simulink model "psc_gfl_parallel"  (R2023b)
settings: Solver=VariableStepAuto  StartTime=0.0  StopTime=1  RelTol=1e-3
values from neighbouring files (symbols this model uses):
  alpha_c = 2*pi*400    (= 2513.27412287)    [init.m]    (also in init_psc_parallel.m)
  f_sw = 10e3    (= 10000)    [init.m]    (also in init_psc_parallel.m)
  kpp = 3/2 * K^(-2)    (= 1.5)    [init.m]    (also in init_psc_parallel.m)
  L_f = 1e-3    (= 0.001)    [init.m]    (also in init_psc_parallel.m = 0.01)
  L_f1 = L_f    (= 0.001)    [init.m]    (also in init_psc_parallel.m = 0.01)
  L_f2 = L_f    (= 0.001)    [init.m]    (also in init_psc_parallel.m = 0.01)
  L_g = 2.5e-3    (= 0.0025)    [init.m]    (also in init_psc_parallel.m)
  R_a = 0.6    [init.m]    (also in init_psc_parallel.m = 0.32)
  R_L = 20    [init.m]    (also in init_psc_parallel.m)
  T_s = 1/(2*f_sw)    (= 5e-05)    [init.m]    (also in init_psc_parallel.m)
  U_dc = 48    [init.m]    (also in init_psc_parallel.m)
  u_gN = 24    [init.m]    (also in init_psc_parallel.m)
  w0_pll = 2*pi*20    (= 125.663706144)    [init.m]    (also in init_psc_parallel.m)
  w_b = 0.1*w_g    (= 31.4159265359)    [init.m]    (also in init_psc_parallel.m)
  w_g = 2*pi*50    (= 314.159265359)    [init.m]    (also in init_psc_parallel.m; psc_matlab.m = (P_ref - P)*K_p + w_1)
libraries: simulink x2
settings Model: Creator=maatt  LastModifiedBy=chowd
settings DataIOCC: ReturnWorkspaceOutputs=off

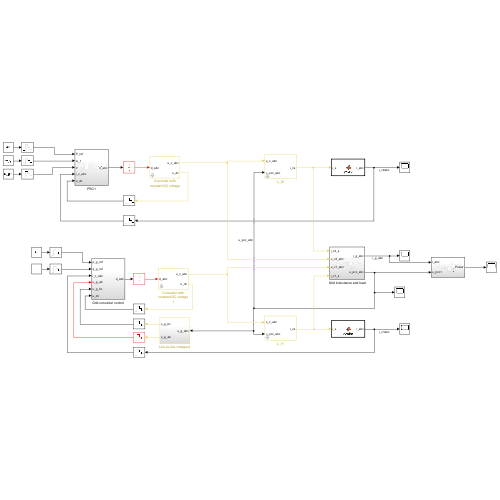
[thumbnail: Simulink's stored preview of the top-level diagram]
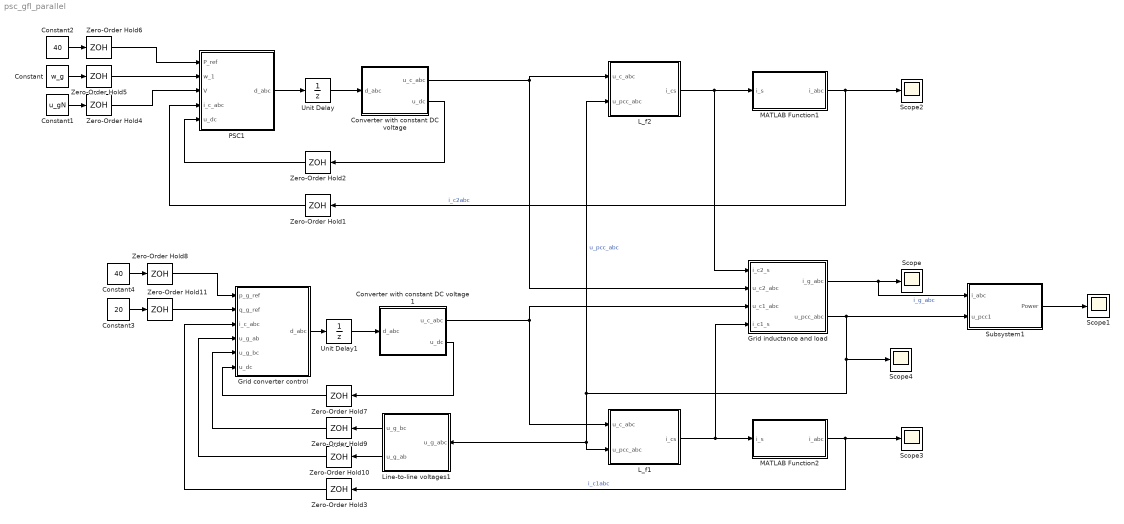
== system psc_gfl_parallel ==
  Constant : Constant  Value=w_g
  Constant1 : Constant  Value=u_gN
  Constant2 : Constant  Value=40  SampleTime=T_s
  Constant3 : Constant  Value=20  SampleTime=T_s
  Constant4 : Constant  Value=40  SampleTime=T_s
  "Converter with constant DC voltage " : Subsystem  mask{f_sw=f_sw, u_dc=U_dc}
      mask prompts: f_sw "Switching frequency (Hz)"; u_dc "DC-bus voltage (V)"
      mask init:
      | T_s = 1/(2*f_sw);
  Converter with constant DC voltage 1 : Subsystem  mask{f_sw=f_sw, u_dc=U_dc}
      mask prompts: f_sw "Switching frequency (Hz)"; u_dc "DC-bus voltage (V)"
      mask init:
      | T_s = 1/(2*f_sw);
  Grid converter control : Subsystem
  Grid inductance and load : Subsystem
  L_f1 : Subsystem  mask{L_f=L_f1, R_f=0}
      mask prompts: L_f "Inductance (H)"; R_f "Series resistance (ohm)"
  L_f2 : Subsystem  mask{L_f=L_f2, R_f=0}
      mask prompts: L_f "Inductance (H)"; R_f "Series resistance (ohm)"
  Line-to-line voltages1 : Subsystem
  MATLAB Function1 : MATLAB Function  TreatAsAtomicUnit=on
  MATLAB Function2 : MATLAB Function  TreatAsAtomicUnit=on
  PSC1 : Subsystem
  Scope{,1..4} (5 alike) : Scope
  Subsystem1 : Subsystem
  Unit Delay : UnitDelay  SampleTime=T_s  HasFrameUpgradeWarning=on
  Unit Delay1 : UnitDelay  SampleTime=T_s  HasFrameUpgradeWarning=on
  Zero-Order Hold{1..11} (11 alike) : ZeroOrderHold  SampleTime=T_s
  wires:
  "Converter with constant DC voltage "/2(u_dc) -> Zero-Order Hold2/1
  Constant2/1 -> Zero-Order Hold6/1
  Constant/1 -> Zero-Order Hold5/1
  Constant1/1 -> Zero-Order Hold4/1
  Unit Delay/1 -> "Converter with constant DC voltage "/1(d_abc)
  Zero-Order Hold1/1 -> PSC1/4(i_c_abc)
  Zero-Order Hold4/1 -> PSC1/3(V)
  Zero-Order Hold5/1 -> PSC1/2(w_1)
  Zero-Order Hold6/1 -> PSC1/1(P_ref)
  Zero-Order Hold2/1 -> PSC1/5(u_dc)
  PSC1/1(d_abc) -> Unit Delay/1
  Line-to-line voltages1/2(u_g_ab) -> Zero-Order Hold10/1
  Converter with constant DC voltage 1/2(u_dc) -> Zero-Order Hold7/1
  Line-to-line voltages1/1(u_g_bc) -> Zero-Order Hold9/1
  Constant3/1 -> Zero-Order Hold11/1
  Zero-Order Hold3/1 -> Grid converter control/3(i_c_abc)
  Zero-Order Hold11/1 -> Grid converter control/2(q_g_ref)
  Zero-Order Hold8/1 -> Grid converter control/1(p_g_ref)
  Unit Delay1/1 -> Converter with constant DC voltage 1/1(d_abc)
  Zero-Order Hold9/1 -> Grid converter control/5(u_g_bc)
  Grid converter control/1(d_abc) -> Unit Delay1/1
  Zero-Order Hold7/1 -> Grid converter control/6(u_dc)
  Zero-Order Hold10/1 -> Grid converter control/4(u_g_ab)
  Constant4/1 -> Zero-Order Hold8/1
  Subsystem1/1(Power) -> Scope1/1
  Grid inductance and load/1(i_g_abc) -> Subsystem1/1(i_abc), Scope/1  "i_g_abc"
  MATLAB Function1/1(i_abc) -> Scope2/1, Zero-Order Hold1/1  "i_c2abc"
  Grid inductance and load/2(u_pcc_abc) -> Scope4/1, L_f2/2(u_pcc_abc), Line-to-line voltages1/1(u_g_abc), L_f1/2(u_pcc_abc), Subsystem1/2(u_pcc1)  "u_pcc_abc"
  L_f2/1(i_cs) -> MATLAB Function1/1(i_s), Grid inductance and load/1(i_c2_s)
  L_f1/1(i_cs) -> Grid inductance and load/4(i_c1_s), MATLAB Function2/1(i_s)
  MATLAB Function2/1(i_abc) -> Zero-Order Hold3/1, Scope3/1  "i_c1abc"
  "Converter with constant DC voltage "/1(u_c_abc) -> L_f2/1(u_c_abc), Grid inductance and load/2(u_c2_abc)
  Converter with constant DC voltage 1/1(u_c_abc) -> L_f1/1(u_c_abc), Grid inductance and load/3(u_c1_abc)

== system psc_gfl_parallel/Converter with constant DC voltage  ==
  note: Voltages u_c_abc = [u_c_aN; u_c_bN; u_c_cN] are the inverter
      | output voltages with respect to the negative DC bus.
  d_abc : Inport
  Constant : Constant  Value=u_dc
  Product : Product
  Relational Operator : RelationalOperator  Operator=>  OutDataTypeStr='double'  InputSameDT=off
  Repeating Sequence : simulink/Sources/Repeating Sequence  rep_seq_t=[0 1 2]*T_s  rep_seq_y=[1 0 1]
  u_c_abc : Outport
  u_dc : Outport  Port=2
  wires:
  Repeating Sequence/1 -> Relational Operator/2
  d_abc/1 -> Relational Operator/1
  Product/1 -> u_c_abc/1
  Relational Operator/1 -> Product/1  "q_abc"
  Constant/1 -> Product/2, u_dc/1

== system psc_gfl_parallel/Converter with constant DC voltage 1 ==
  note: Voltages u_c_abc = [u_c_aN; u_c_bN; u_c_cN] are the inverter
      | output voltages with respect to the negative DC bus.
  d_abc : Inport
  Constant : Constant  Value=u_dc
  Product : Product
  Relational Operator : RelationalOperator  Operator=>  OutDataTypeStr='double'  InputSameDT=off
  Repeating Sequence : simulink/Sources/Repeating Sequence  rep_seq_t=[0 1 2]*T_s  rep_seq_y=[1 0 1]
  u_c_abc : Outport
  u_dc : Outport  Port=2
  wires:
  Repeating Sequence/1 -> Relational Operator/2
  d_abc/1 -> Relational Operator/1
  Product/1 -> u_c_abc/1
  Relational Operator/1 -> Product/1  "q_abc"
  Constant/1 -> Product/2, u_dc/1

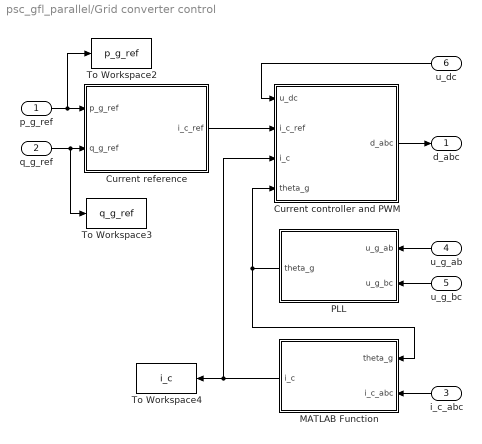
== system psc_gfl_parallel/Grid converter control ==
  p_g_ref : Inport
  q_g_ref : Inport  Port=2
  i_c_abc : Inport  Port=3
  u_g_ab : Inport  Port=4
  u_g_bc : Inport  Port=5
  u_dc : Inport  Port=6
  Current controller and PWM : Subsystem
  Current reference : MATLAB Function  TreatAsAtomicUnit=on
  MATLAB Function : MATLAB Function  TreatAsAtomicUnit=on
  PLL : Subsystem
  To Workspace2 : ToWorkspace  VariableName=p_g_ref  SaveFormat=Timeseries  SampleTime=-1
  To Workspace3 : ToWorkspace  VariableName=q_g_ref  SaveFormat=Timeseries  SampleTime=-1
  To Workspace4 : ToWorkspace  VariableName=i_c  SaveFormat=Timeseries  SampleTime=-1
  d_abc : Outport
  wires:
  i_c_abc/1 -> MATLAB Function/2(i_c_abc)
  Current controller and PWM/1(d_abc) -> d_abc/1
  Current reference/1(i_c_ref) -> Current controller and PWM/2(i_c_ref)
  MATLAB Function/1(i_c) -> To Workspace4/1, Current controller and PWM/3(i_c)
  q_g_ref/1 -> To Workspace3/1, Current reference/2(q_g_ref)
  p_g_ref/1 -> To Workspace2/1, Current reference/1(p_g_ref)
  u_g_bc/1 -> PLL/2(u_g_bc)
  u_g_ab/1 -> PLL/1(u_g_ab)
  PLL/1(theta_g) -> MATLAB Function/1(theta_g), Current controller and PWM/4(theta_g)
  u_dc/1 -> Current controller and PWM/1(u_dc)

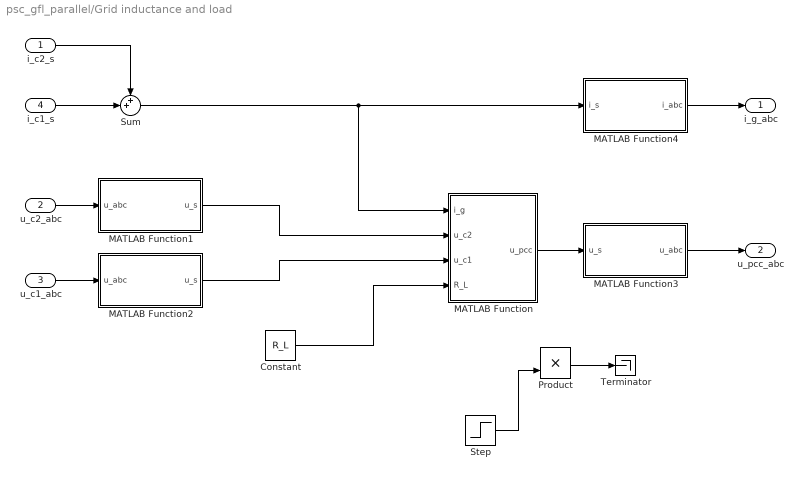
== system psc_gfl_parallel/Grid inductance and load ==
  i_c2_s : Inport
  u_c2_abc : Inport  Port=2
  u_c1_abc : Inport  Port=3
  i_c1_s : Inport  Port=4
  Constant : Constant  Value=R_L  SampleTime=T_s
  MATLAB Function : MATLAB Function  TreatAsAtomicUnit=on
  MATLAB Function1 : MATLAB Function  TreatAsAtomicUnit=on
  MATLAB Function2 : MATLAB Function  TreatAsAtomicUnit=on
  MATLAB Function3 : MATLAB Function  TreatAsAtomicUnit=on
  MATLAB Function4 : MATLAB Function  TreatAsAtomicUnit=on
  Product : Product
  Step : Step  Time=.06  Before=1  After=0.5  SampleTime=T_s
  Sum : Sum  Inputs=++|
  Terminator : Terminator
  i_g_abc : Outport
  u_pcc_abc : Outport  Port=2
  wires:
  Sum/1 -> MATLAB Function4/1(i_s), MATLAB Function/1(i_g)
  i_c2_s/1 -> Sum/1
  i_c1_s/1 -> Sum/2
  u_c2_abc/1 -> MATLAB Function1/1(u_abc)
  u_c1_abc/1 -> MATLAB Function2/1(u_abc)
  MATLAB Function1/1(u_s) -> MATLAB Function/2(u_c2)
  MATLAB Function2/1(u_s) -> MATLAB Function/3(u_c1)
  MATLAB Function/1(u_pcc) -> MATLAB Function3/1(u_s)
  MATLAB Function3/1(u_abc) -> u_pcc_abc/1
  MATLAB Function4/1(i_abc) -> i_g_abc/1
  ? -> Product/1
  Step/1 -> Product/2
  Constant/1 -> MATLAB Function/4(R_L)
  Product/1 -> Terminator/1

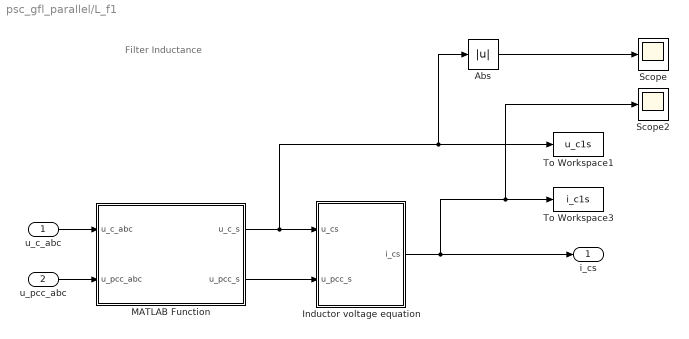
== system psc_gfl_parallel/L_f1 ==
  note: Filter Inductance
  u_c_abc : Inport
  u_pcc_abc : Inport  Port=2
  Abs : Abs  SaturateOnIntegerOverflow=off
  Inductor voltage equation : Subsystem
  MATLAB Function : MATLAB Function  TreatAsAtomicUnit=on
  Scope : Scope
  Scope2 : Scope
  To Workspace1 : ToWorkspace  VariableName=u_c1s  SaveFormat=Timeseries
  To Workspace3 : ToWorkspace  VariableName=i_c1s  SaveFormat=Timeseries
  i_cs : Outport
  wires:
  Abs/1 -> Scope/1
  Inductor voltage equation/1(i_cs) -> i_cs/1, Scope2/1, To Workspace3/1
  MATLAB Function/1(u_c_s) -> Inductor voltage equation/1(u_cs), To Workspace1/1, Abs/1
  u_c_abc/1 -> MATLAB Function/1(u_c_abc)
  MATLAB Function/2(u_pcc_s) -> Inductor voltage equation/2(u_pcc_s)
  u_pcc_abc/1 -> MATLAB Function/2(u_pcc_abc)

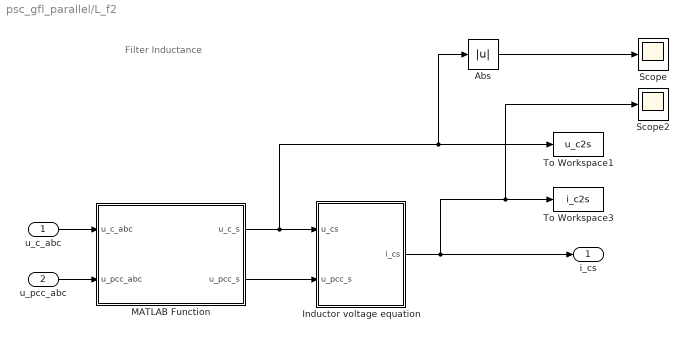
== system psc_gfl_parallel/L_f2 ==
  note: Filter Inductance
  u_c_abc : Inport
  u_pcc_abc : Inport  Port=2
  Abs : Abs  SaturateOnIntegerOverflow=off
  Inductor voltage equation : Subsystem
  MATLAB Function : MATLAB Function  TreatAsAtomicUnit=on
  Scope : Scope
  Scope2 : Scope
  To Workspace1 : ToWorkspace  VariableName=u_c2s  SaveFormat=Timeseries
  To Workspace3 : ToWorkspace  VariableName=i_c2s  SaveFormat=Timeseries
  i_cs : Outport
  wires:
  Abs/1 -> Scope/1
  Inductor voltage equation/1(i_cs) -> i_cs/1, Scope2/1, To Workspace3/1
  MATLAB Function/1(u_c_s) -> Inductor voltage equation/1(u_cs), To Workspace1/1, Abs/1
  u_c_abc/1 -> MATLAB Function/1(u_c_abc)
  MATLAB Function/2(u_pcc_s) -> Inductor voltage equation/2(u_pcc_s)
  u_pcc_abc/1 -> MATLAB Function/2(u_pcc_abc)

== system psc_gfl_parallel/Line-to-line voltages1 ==
  u_g_abc : Inport
  MATLAB Function : MATLAB Function  TreatAsAtomicUnit=on
  u_g_bc : Outport
  u_g_ab : Outport  Port=2
  wires:
  u_g_abc/1 -> MATLAB Function/1(u_abc)
  MATLAB Function/1(u_ab) -> u_g_ab/1
  MATLAB Function/2(u_bc) -> u_g_bc/1

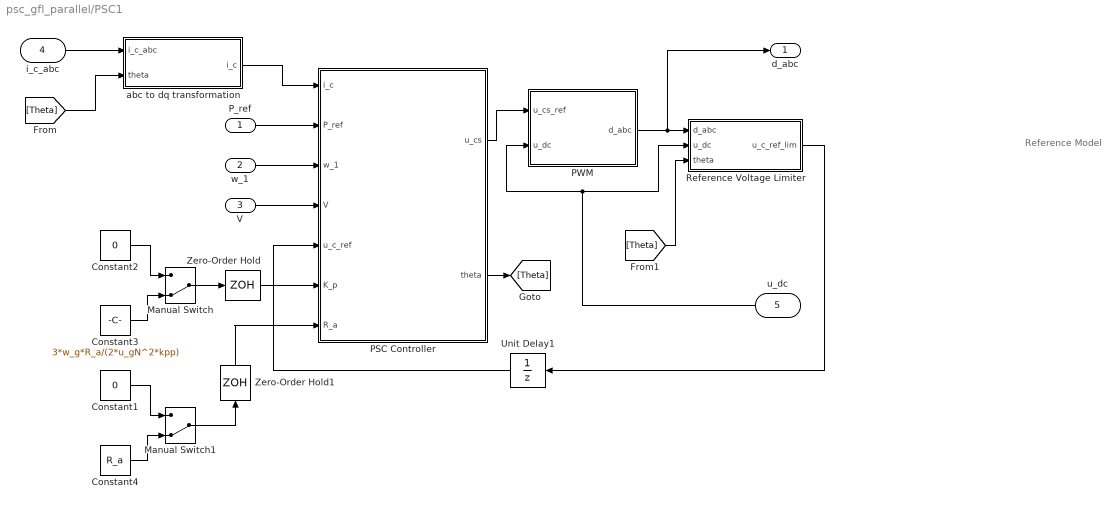
== system psc_gfl_parallel/PSC1 ==
  note: Reference Model
  P_ref : Inport
  w_1 : Inport  Port=2
  V : Inport  Port=3
  i_c_abc : Inport  Port=4
  u_dc : Inport  Port=5
  Constant1 : Constant  Value=0  SampleTime=T_s
  Constant2 : Constant  Value=0  SampleTime=T_s
  Constant3 : Constant  Value=3*w_g*R_a/(2*u_gN^2*kpp)  SampleTime=T_s
  Constant4 : Constant  Value=R_a  SampleTime=T_s
  Manual Switch : ManualSwitch  CurrentSetting=0
  Manual Switch1 : ManualSwitch  CurrentSetting=0
  PSC Controller : Subsystem
  PWM : Subsystem
  Reference Voltage Limiter : Subsystem
  Unit Delay1 : UnitDelay  SampleTime=-1  HasFrameUpgradeWarning=on
  Zero-Order Hold : ZeroOrderHold  SampleTime=T_s
  Zero-Order Hold1 : ZeroOrderHold  SampleTime=T_s
  abc to dq transformation : MATLAB Function  TreatAsAtomicUnit=on
  d_abc : Outport
  wires:
  i_c_abc/1 -> abc to dq transformation/1(i_c_abc)
  [Theta] -> abc to dq transformation/2(theta)
  u_dc/1 -> PWM/2(u_dc), Reference Voltage Limiter/2(u_dc)
  Reference Voltage Limiter/1(u_c_ref_lim) -> Unit Delay1/1
  w_1/1 -> PSC Controller/3(w_1)
  PWM/1(d_abc) -> d_abc/1, Reference Voltage Limiter/1(d_abc)
  [Theta] -> Reference Voltage Limiter/3(theta)
  Unit Delay1/1 -> PSC Controller/5(u_c_ref)
  abc to dq transformation/1(i_c) -> PSC Controller/1(i_c)
  P_ref/1 -> PSC Controller/2(P_ref)
  V/1 -> PSC Controller/4(V)
  PSC Controller/1(u_cs) -> PWM/1(u_cs_ref)
  PSC Controller/2(theta) -> [Theta]
  Constant2/1 -> Manual Switch/1
  Constant3/1 -> Manual Switch/2
  Manual Switch/1 -> Zero-Order Hold/1
  Constant4/1 -> Manual Switch1/2
  Constant1/1 -> Manual Switch1/1
  Manual Switch1/1 -> Zero-Order Hold1/1
  Zero-Order Hold/1 -> PSC Controller/6(K_p)
  Zero-Order Hold1/1 -> PSC Controller/7(R_a)

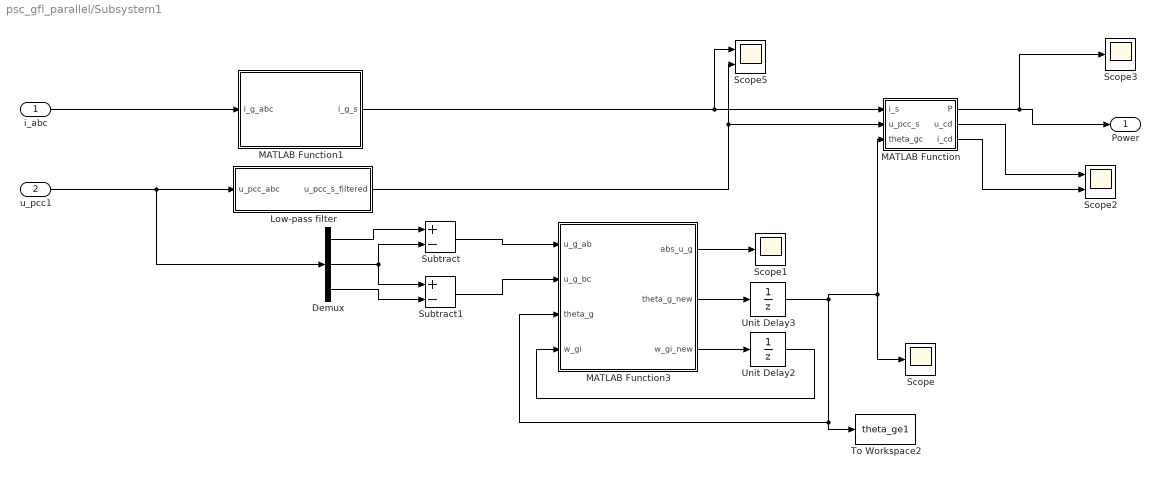
== system psc_gfl_parallel/Subsystem1 ==
  i_abc : Inport
  u_pcc1 : Inport  Port=2
  Demux : Demux  Outputs=3
  Low-pass filter : Subsystem
  MATLAB Function : MATLAB Function  TreatAsAtomicUnit=on
  MATLAB Function1 : MATLAB Function  TreatAsAtomicUnit=on
  MATLAB Function3 : MATLAB Function  TreatAsAtomicUnit=on
  Scope : Scope
  Scope1 : Scope
  Scope2 : Scope  NumInputPorts=2
  Scope3 : Scope
  Scope5 : Scope  NumInputPorts=2
  Subtract : Sum  Inputs=+-
  Subtract1 : Sum  Inputs=+-
  To Workspace2 : ToWorkspace  VariableName=theta_ge1  SaveFormat=Timeseries  SampleTime=-1
  Unit Delay2 : UnitDelay  InitialCondition=w_g  SampleTime=-1  HasFrameUpgradeWarning=on
  Unit Delay3 : UnitDelay  SampleTime=-1  HasFrameUpgradeWarning=on
  Power : Outport
  wires:
  MATLAB Function/1(P) -> Scope3/1, Power/1
  i_abc/1 -> MATLAB Function1/1(i_g_abc)
  Low-pass filter/1(u_pcc_s_filtered) -> Scope5/2, MATLAB Function/2(u_pcc_s)
  Unit Delay2/1 -> MATLAB Function3/4(w_gi)
  MATLAB Function3/2(theta_g_new) -> Unit Delay3/1
  Unit Delay3/1 -> Scope/1, MATLAB Function/3(theta_gc), To Workspace2/1, MATLAB Function3/3(theta_g)
  MATLAB Function3/3(w_gi_new) -> Unit Delay2/1
  u_pcc1/1 -> Demux/1, Low-pass filter/1(u_pcc_abc)
  MATLAB Function3/1(abs_u_g) -> Scope1/1
  Demux/3 -> Subtract1/2
  Subtract/1 -> MATLAB Function3/1(u_g_ab)
  Demux/1 -> Subtract/1
  Demux/2 -> Subtract/2, Subtract1/1
  Subtract1/1 -> MATLAB Function3/2(u_g_bc)
  MATLAB Function/2(u_cd) -> Scope2/1
  MATLAB Function/3(i_cd) -> Scope2/2
  MATLAB Function1/1(i_g_s) -> Scope5/1, MATLAB Function/1(i_s)

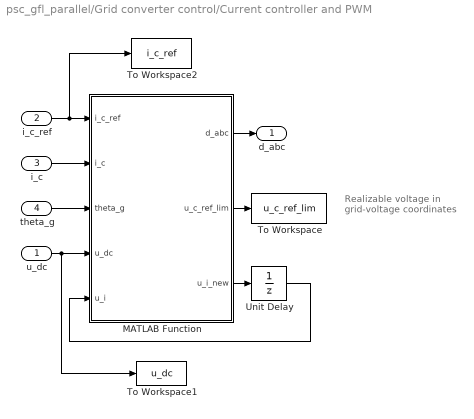
== system psc_gfl_parallel/Grid converter control/Current controller and PWM ==
  note: Realizable voltage
      | in grid-voltage coordinates
  u_dc : Inport
  i_c_ref : Inport  Port=2
  i_c : Inport  Port=3
  theta_g : Inport  Port=4
  MATLAB Function : MATLAB Function  TreatAsAtomicUnit=on
  To Workspace : ToWorkspace  VariableName=u_c_ref_lim  SaveFormat=Timeseries  SampleTime=-1
  To Workspace1 : ToWorkspace  VariableName=u_dc  SaveFormat=Timeseries  SampleTime=-1
  To Workspace2 : ToWorkspace  VariableName=i_c_ref  SaveFormat=Timeseries  SampleTime=-1
  Unit Delay : UnitDelay  InitialCondition=u_gN  SampleTime=-1  HasFrameUpgradeWarning=on
  d_abc : Outport  PortDimensions=3
  wires:
  MATLAB Function/3(u_i_new) -> Unit Delay/1
  i_c_ref/1 -> To Workspace2/1, MATLAB Function/1(i_c_ref)
  i_c/1 -> MATLAB Function/2(i_c)
  Unit Delay/1 -> MATLAB Function/5(u_i)
  MATLAB Function/1(d_abc) -> d_abc/1
  MATLAB Function/2(u_c_ref_lim) -> To Workspace/1
  theta_g/1 -> MATLAB Function/3(theta_g)
  u_dc/1 -> To Workspace1/1, MATLAB Function/4(u_dc)

== system psc_gfl_parallel/Grid converter control/PLL ==
  u_g_ab : Inport
  u_g_bc : Inport  Port=2
  MATLAB Function : MATLAB Function  TreatAsAtomicUnit=on
  To Workspace1 : ToWorkspace  VariableName=theta_ge  SaveFormat=Timeseries  SampleTime=-1
  To Workspace4 : ToWorkspace  VariableName=abs_u_g  SaveFormat=Timeseries  SampleTime=-1
  Unit Delay : UnitDelay  InitialCondition=w_g  SampleTime=-1  HasFrameUpgradeWarning=on
  Unit Delay1 : UnitDelay  SampleTime=-1  HasFrameUpgradeWarning=on
  theta_g : Outport
  wires:
  u_g_bc/1 -> MATLAB Function/2(u_g_bc)
  u_g_ab/1 -> MATLAB Function/1(u_g_ab)
  MATLAB Function/1(abs_u_g) -> To Workspace4/1
  MATLAB Function/3(w_gi_new) -> Unit Delay/1
  MATLAB Function/2(theta_g_new) -> Unit Delay1/1
  Unit Delay1/1 -> MATLAB Function/3(theta_g), To Workspace1/1, theta_g/1
  Unit Delay/1 -> MATLAB Function/4(w_gi)

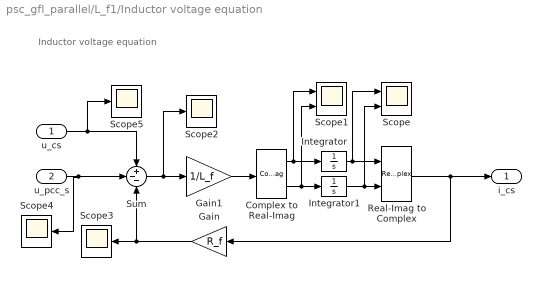
== system psc_gfl_parallel/L_f1/Inductor voltage equation ==
  note: Inductor voltage equation
  u_cs : Inport
  u_pcc_s : Inport  Port=2
  Complex to Real-Imag : ComplexToRealImag
  Gain : Gain  Gain=R_f
  Gain1 : Gain  Gain=1/L_f
  Integrator : Integrator
  Integrator1 : Integrator
  Real-Imag to Complex : RealImagToComplex
  Scope : Scope  NumInputPorts=2
  Scope1 : Scope  NumInputPorts=2
  Scope{2..5} (4 alike) : Scope
  Sum : Sum  Inputs=+--
  i_cs : Outport
  wires:
  Gain/1 -> Scope3/1, Sum/3
  Real-Imag to Complex/1 -> i_cs/1, Gain/1
  Integrator1/1 -> Real-Imag to Complex/2, Scope/2
  Integrator/1 -> Real-Imag to Complex/1, Scope/1
  Complex to Real-Imag/2 -> Integrator1/1, Scope1/2
  Complex to Real-Imag/1 -> Integrator/1, Scope1/1
  Gain1/1 -> Complex to Real-Imag/1
  Sum/1 -> Scope2/1, Gain1/1
  u_pcc_s/1 -> Scope4/1, Sum/2
  u_cs/1 -> Scope5/1, Sum/1

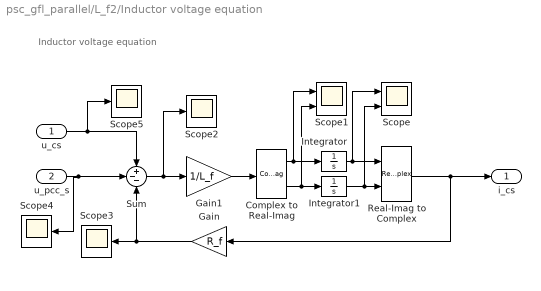
== system psc_gfl_parallel/L_f2/Inductor voltage equation ==
  note: Inductor voltage equation
  u_cs : Inport
  u_pcc_s : Inport  Port=2
  Complex to Real-Imag : ComplexToRealImag
  Gain : Gain  Gain=R_f
  Gain1 : Gain  Gain=1/L_f
  Integrator : Integrator
  Integrator1 : Integrator
  Real-Imag to Complex : RealImagToComplex
  Scope : Scope  NumInputPorts=2
  Scope1 : Scope  NumInputPorts=2
  Scope{2..5} (4 alike) : Scope
  Sum : Sum  Inputs=+--
  i_cs : Outport
  wires:
  Gain/1 -> Scope3/1, Sum/3
  Real-Imag to Complex/1 -> i_cs/1, Gain/1
  Integrator1/1 -> Real-Imag to Complex/2, Scope/2
  Integrator/1 -> Real-Imag to Complex/1, Scope/1
  Complex to Real-Imag/2 -> Integrator1/1, Scope1/2
  Complex to Real-Imag/1 -> Integrator/1, Scope1/1
  Gain1/1 -> Complex to Real-Imag/1
  Sum/1 -> Scope2/1, Gain1/1
  u_pcc_s/1 -> Scope4/1, Sum/2
  u_cs/1 -> Scope5/1, Sum/1

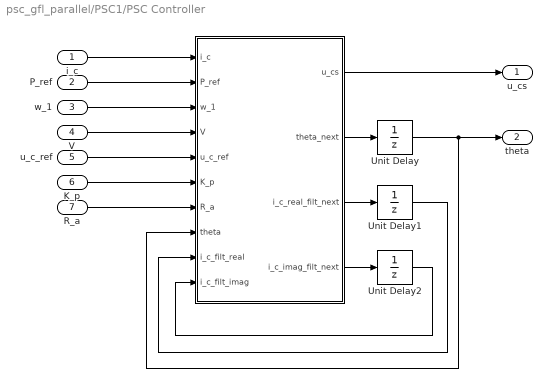
== system psc_gfl_parallel/PSC1/PSC Controller ==
  i_c : Inport
  P_ref : Inport  Port=2
  w_1 : Inport  Port=3
  V : Inport  Port=4
  u_c_ref : Inport  Port=5
  K_p : Inport  Port=6
  R_a : Inport  Port=7
  " " : MATLAB Function  TreatAsAtomicUnit=on
  Unit Delay : UnitDelay  SampleTime=-1  HasFrameUpgradeWarning=on
  Unit Delay1 : UnitDelay  SampleTime=-1  HasFrameUpgradeWarning=on
  Unit Delay2 : UnitDelay  SampleTime=-1  HasFrameUpgradeWarning=on
  u_cs : Outport
  theta : Outport  Port=2
  wires:
  " "/1(u_cs) -> u_cs/1
  " "/2(theta_next) -> Unit Delay/1
  V/1 -> " "/4(V)
  P_ref/1 -> " "/2(P_ref)
  i_c/1 -> " "/1(i_c)
  w_1/1 -> " "/3(w_1)
  u_c_ref/1 -> " "/5(u_c_ref)
  Unit Delay/1 -> theta/1, " "/8(theta)
  " "/3(i_c_real_filt_next) -> Unit Delay1/1
  " "/4(i_c_imag_filt_next) -> Unit Delay2/1
  Unit Delay1/1 -> " "/9(i_c_filt_real)
  Unit Delay2/1 -> " "/10(i_c_filt_imag)
  K_p/1 -> " "/6(K_p)
  R_a/1 -> " "/7(R_a)

== system psc_gfl_parallel/PSC1/PWM ==
  u_cs_ref : Inport
  u_dc : Inport  Port=2
  MATLAB Function : MATLAB Function  TreatAsAtomicUnit=on
  d_abc : Outport
  wires:
  u_cs_ref/1 -> MATLAB Function/1(u_cs_ref)
  u_dc/1 -> MATLAB Function/2(u_dc)
  MATLAB Function/1(d_abc) -> d_abc/1

== system psc_gfl_parallel/PSC1/Reference Voltage Limiter ==
  d_abc : Inport
  u_dc : Inport  Port=2
  theta : Inport  Port=3
  MATLAB Function : MATLAB Function  TreatAsAtomicUnit=on
  u_c_ref_lim : Outport
  wires:
  d_abc/1 -> MATLAB Function/1(d_abc)
  theta/1 -> MATLAB Function/3(theta)
  MATLAB Function/1(u_c_ref_lim) -> u_c_ref_lim/1
  u_dc/1 -> MATLAB Function/2(u_dc)

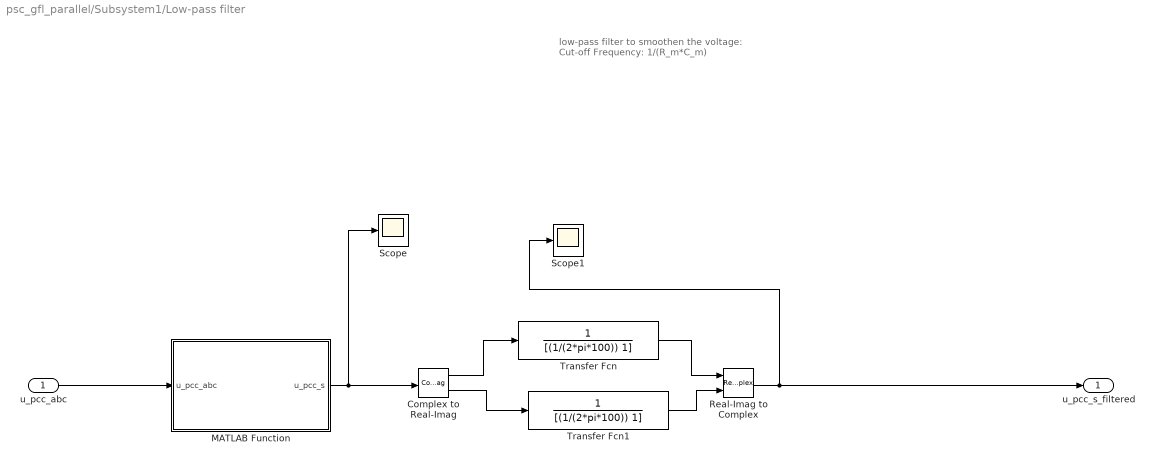
== system psc_gfl_parallel/Subsystem1/Low-pass filter ==
  note: low-pass filter to smoothen the voltage:
      | Cut-off Frequency: 1/(R_m*C_m)
  u_pcc_abc : Inport
  Complex to Real-Imag : ComplexToRealImag
  MATLAB Function : MATLAB Function  TreatAsAtomicUnit=on
  Real-Imag to Complex : RealImagToComplex
  Scope : Scope
  Scope1 : Scope
  Transfer Fcn : TransferFcn  Denominator=[(1/(2*pi*100)) 1]
  Transfer Fcn1 : TransferFcn  Denominator=[(1/(2*pi*100)) 1]
  u_pcc_s_filtered : Outport
  wires:
  Complex to Real-Imag/2 -> Transfer Fcn1/1
  Transfer Fcn/1 -> Real-Imag to Complex/1
  u_pcc_abc/1 -> MATLAB Function/1(u_pcc_abc)
  MATLAB Function/1(u_pcc_s) -> Scope/1, Complex to Real-Imag/1
  Complex to Real-Imag/1 -> Transfer Fcn/1
  Real-Imag to Complex/1 -> Scope1/1, u_pcc_s_filtered/1
  Transfer Fcn1/1 -> Real-Imag to Complex/2

== matlab function psc_gfl_parallel/L_f2/MATLAB Function ==
  data: u_c_abc input; u_pcc_abc input; u_c_s output; u_pcc_s output
function [u_c_s, u_pcc_s] = abc2s(u_c_abc, u_pcc_abc)

% Space Vector Transformation of converter and pcc voltage
u_c_s = 2/3*(u_c_abc(1) + u_c_abc(2)*exp(1j*2*pi/3) + u_c_abc(3)*exp(1j*4*pi/3));

u_pcc_s = 2/3*(u_pcc_abc(1) + u_pcc_abc(2)*exp(1j*2*pi/3) + u_pcc_abc(3)*exp(1j*4*pi/3));

== matlab function psc_gfl_parallel/PSC1/Reference Voltage Limiter/MATLAB Function ==
  data: d_abc input; u_dc input; u_c_ref_lim output; theta input; w_g parameter; T_s parameter
function u_c_ref_lim = ref_lim(d_abc, u_dc, theta, w_g, T_s)

% % Realized voltage vector is calculated from the clamped duty ratios.
% % If the PWM does not saturate, u_c_ref_lim = u_c_ref holds. The realized
% % voltage vector is needed, e.g., for the current-controller antiwindup.
u_cs_ref_lim = 2/3*(d_abc(1) + d_abc(2)*exp(1j*2*pi/3) ...
    + d_abc(3)*exp(1j*4*pi/3))*u_dc;

% % In estimated rotor flux coordinates
u_c_ref_lim = exp(-1j*(theta + 1.5 * w_g * T_s))*u_cs_ref_lim;

== matlab function psc_gfl_parallel/PSC1/abc to dq transformation ==
  data: i_c output; i_c_abc input; theta input
function i_c = abc2dq(i_c_abc, theta)

% Space Vector Transformation (abc to alpha-beta)
i_cs = 2/3 * (i_c_abc(1) + i_c_abc(2)*exp(1j*2*pi/3) ... 
    + i_c_abc(3)*exp(1j*4*pi/3));

% Coordinate Transformation (Alpha-beta to dq)
i_c = i_cs * exp(-1j*theta);

== matlab function psc_gfl_parallel/Grid converter control/MATLAB Function ==
  data: theta_g input size=1; i_c_abc input size=3; i_c output size=1
function i_c = abc2dq(theta_g, i_c_abc)

% Space-vector transformation
i_cs = 2/3*(i_c_abc(1) + i_c_abc(2)*exp(1j*2*pi/3) ...
    + i_c_abc(3)*exp(1j*4*pi/3));

% Coordinate transformation
i_c = i_cs*exp(-1j*theta_g);

== matlab function psc_gfl_parallel/Grid converter control/PLL/MATLAB Function ==
  data: u_g_ab input size=1; u_g_bc input size=1; theta_g input; w_gi input; u_gN parameter; w0_pll parameter; abs_u_g output size=1; theta_g_new output; w_gi_new output; T_s parameter
function [abs_u_g, theta_g_new, w_gi_new] = pll(u_g_ab, u_g_bc, ...
    theta_g, w_gi, u_gN, w0_pll, T_s)

% Parameters 
% (Tuning of the PLL is analogous to that of the DC-voltage controller.)
zeta = 1;   % Damping ratio
k_p = 2*zeta*w0_pll/u_gN; 
k_i = w0_pll^2/u_gN;

% Space-vector transformation from line-to-line components
u_gs = 2/3*(u_g_ab - u_g_bc*exp(1j*4*pi/3));

% Coordinate transformation to the "estimated" grid coordinates
u_g = u_gs*exp(-1j*theta_g);

% Error signal, which is drive to zero by the PLL
u_gq = imag(u_g);

w_g = k_p*u_gq + w_gi;

% Update the integral state
w_gi_new = w_gi + T_s*k_i*u_gq;

% Update the grid-voltage angle
theta_g_new = theta_g + T_s*w_g;
while(theta_g_new > pi)
    theta_g_new = theta_g_new - 2*pi;
end
while(theta_g_new < -pi)
    theta_g_new = theta_g_new + 2*pi;
end

% Absolute value of the grid-voltage vector
abs_u_g = abs(u_g);

== matlab function psc_gfl_parallel/MATLAB Function1 ==
  data: i_s input size=1; i_abc output size=3
function i_abc = s2abc(i_s)

% Inverse space-vector transformation
i_abc = real([1; exp(-1j*2*pi/3); exp(-1j*4*pi/3)]*i_s);

== matlab function psc_gfl_parallel/MATLAB Function2 ==
  data: i_s input size=1; i_abc output size=3
function i_abc = s2abc(i_s)

% Inverse space-vector transformation
i_abc = real([1; exp(-1j*2*pi/3); exp(-1j*4*pi/3)]*i_s);

== matlab function psc_gfl_parallel/Subsystem1/Low-pass filter/MATLAB Function ==
  data: u_pcc_abc input; u_pcc_s output
function u_pcc_s  = abc2s(u_pcc_abc)

% Space Vector Transformation of converter and pcc voltage
u_pcc_s = 2/3*(u_pcc_abc(1) + u_pcc_abc(2)*exp(1j*2*pi/3) + u_pcc_abc(3)*exp(1j*4*pi/3));

== matlab function psc_gfl_parallel/Subsystem1/MATLAB Function ==
  data: i_s input; u_pcc_s input; P output; theta_gc input; u_cd output; i_cd output
function [P,u_cd,i_cd] = fcn(i_s, u_pcc_s, theta_gc)
% Reference in stator coordinates
   % Compensation for discrete-time delays
u_cd = (u_pcc_s.*exp(-1j*theta_gc));
i_cd = (i_s.*exp(-1j*theta_gc));
P = 3/2*real((u_cd)*conj(i_cd));

== matlab function psc_gfl_parallel/Subsystem1/MATLAB Function1 ==
  data: i_g_abc input; i_g_s output
function i_g_s  = abc2s(i_g_abc)

% Space Vector Transformation of converter and pcc voltage
i_g_s = 2/3*(i_g_abc(1) + i_g_abc(2)*exp(1j*2*pi/3) + i_g_abc(3)*exp(1j*4*pi/3));

== matlab function psc_gfl_parallel/Line-to-line voltages1/MATLAB Function ==
  data: u_abc input; u_ab output; u_bc output
function [u_ab, u_bc] = ln2ll(u_abc)

u_ab = u_abc(1) - u_abc(2);
u_bc = u_abc(2) - u_abc(3);

== matlab function psc_gfl_parallel/Grid inductance and load/MATLAB Function1 ==
  data: u_abc input size=3; u_s output size=1
function u_s = abc2s(u_abc)

% Space-vector transformation
u_s = 2/3*(u_abc(1) + u_abc(2)*exp(1j*2*pi/3) + u_abc(3)*exp(1j*4*pi/3));

== matlab function psc_gfl_parallel/Grid inductance and load/MATLAB Function2 ==
  data: u_abc input size=3; u_s output size=1
function u_s = abc2s(u_abc)

% Space-vector transformation
u_s = 2/3*(u_abc(1) + u_abc(2)*exp(1j*2*pi/3) + u_abc(3)*exp(1j*4*pi/3));

== matlab function psc_gfl_parallel/Grid inductance and load/MATLAB Function3 ==
  data: u_s input size=1; u_abc output size=3
function u_abc = s2abc(u_s)

% Inverse space-vector transformation
u_abc = real([1; exp(-1j*2*pi/3); exp(-1j*4*pi/3)]*u_s);

== matlab function psc_gfl_parallel/Grid inductance and load/MATLAB Function4 ==
  data: i_s input size=1; i_abc output size=3
function i_abc = s2abc(i_s)

% Inverse space-vector transformation
i_abc = real([1; exp(-1j*2*pi/3); exp(-1j*4*pi/3)]*i_s);

== matlab function psc_gfl_parallel/Subsystem1/MATLAB Function3 ==
  data: abs_u_g output; u_g_ab input size=1; u_g_bc input size=1; theta_g input; w_gi input; u_gN parameter; w0_pll parameter; theta_g_new output; w_gi_new output; T_s parameter
function [abs_u_g, theta_g_new, w_gi_new] = pll(u_g_ab, u_g_bc, theta_g, w_gi, u_gN, w0_pll, T_s)
% Parameters 
% (Tuning of the PLL is analogous to that of the DC-voltage controller.)
zeta = 1;   % Damping ratio
k_p = 2*zeta*w0_pll/u_gN; 
k_i = w0_pll^2/u_gN;

% Space-vector transformation from line-to-line components
u_a = (2*u_g_ab+u_g_bc)/3;
u_b = (-u_g_ab+u_g_bc)/3;
u_c = (-u_g_ab-2*u_g_bc)/3;
u_gs = 2/3*(u_a + u_b*exp(1j*2*pi/3) + u_c*exp(1j*4*pi/3));


% Coordinate transformation to the "estimated" grid coordinates
u_g = u_gs*exp(-1i*theta_g);

% Error signal, which is drive to zero by the PLL
u_gq = imag(u_g);

w_g = k_p*u_gq + w_gi;

% Update the integral state
w_gi_new = w_gi + T_s*k_i*u_gq;

% Update the grid-voltage angle
theta_g_new = theta_g + T_s*w_g;
while(theta_g_new > pi)
    theta_g_new = theta_g_new - 2*pi;
end
while(theta_g_new < -pi)
    theta_g_new = theta_g_new + 2*pi;
end

% Absolute value of the grid-voltage vector
abs_u_g = abs(u_g);

== matlab function psc_gfl_parallel/L_f1/MATLAB Function ==
  data: u_c_abc input; u_pcc_abc input; u_c_s output; u_pcc_s output
function [u_c_s, u_pcc_s] = abc2s(u_c_abc, u_pcc_abc)

% Space Vector Transformation of converter and pcc voltage
u_c_s = 2/3*(u_c_abc(1) + u_c_abc(2)*exp(1j*2*pi/3) + u_c_abc(3)*exp(1j*4*pi/3));

u_pcc_s = 2/3*(u_pcc_abc(1) + u_pcc_abc(2)*exp(1j*2*pi/3) + u_pcc_abc(3)*exp(1j*4*pi/3));

== matlab function psc_gfl_parallel/PSC1/PWM/MATLAB Function ==
  data: d_abc output; u_cs_ref input; u_dc input
function d_abc = PWM(u_cs_ref, u_dc)

%% Symmetrical suboscillation PWM
% Components of the voltage space vector
u_c_alpha_ref = real(u_cs_ref);
u_c_beta_ref  = imag(u_cs_ref);

% Phase-voltage references
u_ca_ref = u_c_alpha_ref;
u_cb_ref = .5*(-u_c_alpha_ref + sqrt(3)*u_c_beta_ref);
u_cc_ref = .5*(-u_c_alpha_ref - sqrt(3)*u_c_beta_ref);

% Vector of phase-voltage references
u_c_abc_ref = [u_ca_ref; u_cb_ref; u_cc_ref];

% Symmetrization of the references by adding the zero-sequence voltage
u0 = .5*(max(u_c_abc_ref) + min(u_c_abc_ref));
u_c_abc_ref = u_c_abc_ref - u0;

% Clipping of the reference voltages such that no phase error is caused. 
% If all phase voltage reference are realizable (below u_dc/2), m = 1 holds.
m = max([2*u_c_abc_ref/u_dc; 1]);
u_c_abc_ref = u_c_abc_ref/m;

% Duty cycles, which can be directly used for triangle comparison, 
% if the triangle wave varies between 0...1
d_abc = .5 + u_c_abc_ref/u_dc;

== matlab function psc_gfl_parallel/Grid converter control/Current controller and PWM/MATLAB Function ==
  data: i_c_ref input size=1; i_c input size=1; theta_g input size=1; u_dc input size=1; u_i input size=1; w_g parameter size=1; L_f parameter size=1; alpha_c parameter size=1; T_s parameter size=1; d_abc output size=3; u_c_ref_lim output size=1; u_i_new output size=1
function [d_abc, u_c_ref_lim, u_i_new] = cc(i_c_ref, i_c, ...
    theta_g, u_dc, u_i, w_g, L_f, alpha_c, T_s)

%% Current controller 
% Gains
k_i = alpha_c^2*L_f;                % Integral gain
k_t = alpha_c*L_f;                  % Reference gain
k_p = (2*alpha_c - 1j*w_g)*L_f;     % Proportional gain

% Voltage reference in synchronous coordinates
u_c_ref = k_t*i_c_ref - k_p*i_c + u_i;

% Reference in stator coordinates
theta_gc = theta_g + 1.5*T_s*w_g;   % Compensation for discrete-time delays
u_cs_ref = u_c_ref*exp(1j*theta_gc);

%% Symmetrical suboscillation PWM
% Components of the voltage space vector
u_c_alpha_ref = real(u_cs_ref);
u_c_beta_ref  = imag(u_cs_ref);

% Phase-voltage references
u_ca_ref = u_c_alpha_ref;
u_cb_ref = .5*(-u_c_alpha_ref + sqrt(3)*u_c_beta_ref);
u_cc_ref = .5*(-u_c_alpha_ref - sqrt(3)*u_c_beta_ref);

% Vector of phase-voltage references
u_c_abc_ref = [u_ca_ref; u_cb_ref; u_cc_ref];

% Symmetrization of the references by adding the zero-sequence voltage
u0 = .5*(max(u_c_abc_ref) + min(u_c_abc_ref));
u_c_abc_ref = u_c_abc_ref - u0;

% Clipping of the reference voltages such that no phase error is caused. 
% If all phase voltage reference are realizable (below u_dc/2), m = 1 holds.
m = max([2*u_c_abc_ref/u_dc; 1]);
u_c_abc_ref = u_c_abc_ref/m;

% Duty cycles, which can be directly used for triangle comparison, 
% if the triangle wave varies between 0...1
d_abc = .5 + u_c_abc_ref/u_dc;

% Realized voltage vector is calculated from the clamped duty ratios.
% If the PWM does not saturate, u_c_ref_lim = u_c_ref holds. The realized
% voltage vector is needed, e.g., for the current-controller antiwindup.
u_cs_ref_lim = 2/3*(d_abc(1) + d_abc(2)*exp(1j*2*pi/3) ...
    + d_abc(3)*exp(1j*4*pi/3))*u_dc;
% In estimated rotor flux coordinates
u_c_ref_lim = exp(-1j*theta_gc)*u_cs_ref_lim;  

%% Update the integral state of the current controller 
u_i_new = u_i + T_s*k_i*(i_c_ref - i_c + (u_c_ref_lim - u_c_ref)/k_t);

== matlab function psc_gfl_parallel/Grid converter control/Current reference ==
  data: p_g_ref input; q_g_ref input; i_c_ref output; u_gN parameter size=1
function i_c_ref = curr_ref(p_g_ref, q_g_ref, u_gN)

% Current references in grid-voltage coordinates
i_c_ref = ((2/3)*p_g_ref/u_gN) + 1j*((-2/3)*q_g_ref/u_gN);

== matlab function psc_gfl_parallel/Grid inductance and load/MATLAB Function ==
  data: i_g input; u_pcc output; u_c2 input; L_g parameter; L_f1 parameter; L_f2 parameter; u_c1 input; R_L input
function u_pcc = fcn(i_g, u_c2, L_g, L_f1, L_f2, u_c1, R_L)

u_pcc = (L_g*(u_c1/L_f1+u_c2/L_f2)+R_L*i_g)/(1+L_g/L_f1+L_g/L_f2);

== matlab function psc_gfl_parallel/PSC1/PSC Controller/  ==
  data: i_c input; P_ref input; u_cs output; theta_next output; w_1 input; V input; u_c_ref input; K_p input; R_a input; theta input; i_c_filt_real input; i_c_filt_imag input; T_s parameter; i_c_real_filt_next output; i_c_imag_filt_next output; w_b parameter; kpp parameter
function [u_cs, theta_next, i_c_real_filt_next, i_c_imag_filt_next] = ... 
    PSC(i_c, P_ref, w_1, V, u_c_ref, K_p, R_a, theta, i_c_filt_real, i_c_filt_imag, ... 
    T_s, w_b, kpp)

% Active power calculation
P = kpp*real(u_c_ref*conj(i_c));

% Equation for grid angular frequency
w_g = (P_ref - P)*K_p + w_1;

% Update (integrate) the grid voltage angle
theta_next = theta + T_s * w_g; 

%Limiting theta value -pi <= theta <= pi
if(theta_next > pi)
    theta_next = theta_next - 2*pi;
end
if(theta_next < -pi)
    theta_next = theta_next + 2*pi;
end

% Extracting the real and imaginary values of the complex converter current
i_c_real = real(i_c);
i_c_imag = imag(i_c);

% Applying highpass filter equation to real and imaginary parts of the
% converter current
i_c_real_filt_next =  i_c_filt_real*(1 - w_b*T_s) + i_c_real*(w_b*T_s);
i_c_imag_filt_next =  i_c_filt_imag*(1 - w_b*T_s) + i_c_imag*(w_b*T_s);

% Equation for reference voltage
u_c = V - ((i_c_real - i_c_real_filt_next) + 1j*(i_c_imag - i_c_imag_filt_next)) * R_a;

% Inverse coordinate transformation with discrete time compensation
u_cs = u_c*exp(1j*(theta + 1.5 * T_s * w_1));
